simulink model "foc_model"  (R2020b)
settings: Solver=VariableStepAuto  StartTime=0.0  StopTime=0.08  FixedStep=tsim  RelTol=1e-3
undefined symbols (not defined in the file): denZC_id, denZC_iq, denZC_w, ee_sli_rtmsupport, gcbh, numZC_id, numZC_iq, numZC_w, torque0, Tsc
libraries: fl_lib x32, ee_lib x23, nesl_utility x15, slctrlblks x3, eeDiscretePi x3, eeTransforms x2, eeDqVoltageLimiter x1, eePmsmCurrentReferenceGen x1, simulink x1, eePwmGeneratorTwoLevel x1
(part 1 of 2)
settings Model: Creator=1  LastModifiedBy=ahudobin
settings SimscapeCC: SimscapeLogType=all  SimscapeLogDataHistory=10000

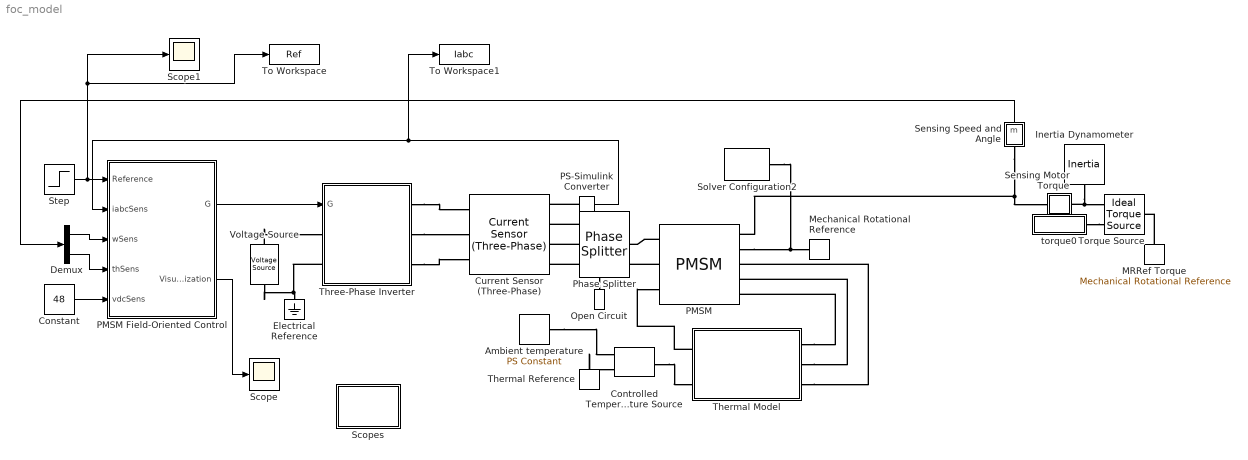
== system foc_model ==
  Ambient temperature : fl_lib/Physical Signals/Sources/PS Constant  constant=298 K
  Constant : Constant  Value=48
  Controlled Temperature Source : fl_lib/Thermal/Thermal Sources/Controlled Temperature Source
  Current Sensor (Three-Phase) : ee_lib/Sensors & Transducers/Current Sensor (Three-Phase)
      settings: InternalSimscapePortConfiguration="{\"Bottom\":[],\"Left\":[{\"id\":\"a1\",\"label\":\"a1\",\"type\":\"foundation.electrical.electrical\"},{\"id\":\"b1\",\"label\":\"b1\",\"type\":\"foundation.electrical.electrical\"},{\"id\":\"c1\",\"label\":\"c1\",\"type\":\"foundation.electrical.electrical\"}],\"Right\":[{\"id\":\"I_output\",\"label\":\"I\",\"type\":\"output\"},{\"id\":\"a2\",\"label\":\"a2\",\"type\":\"foundation.electrical.electrical\"},{\"id\":\"b2\",\"label\":\"b2\",\"type\":\"foundation.electrical.electrical\"},{\"id\":\"c2\",\"label\":\"c2\",\"type\":\"foundation.electrical.electrical\"}],\"Top\":[]}"
  Demux : Demux  Outputs=2
  Electrical Reference : fl_lib/Electrical/Electrical Elements/Electrical Reference
  Inertia Dynamometer : fl_lib/Mechanical/Rotational Elements/Inertia  inertia=1 kg*m^2  num_ports=foundation.enum.numPorts2.one  w_specify=on  w_priority=High  w=0 rpm  w_nominal_specify=off  w_nominal_unit=rad/s  w_nominal_value=1  t_specify=off  t_priority=High  t=0 N*m  t_nominal_specify=off  t_nominal_unit=N*m  t_nominal_value=1
  MRRef Torque : fl_lib/Mechanical/Rotational Elements/Mechanical Rotational Reference
  Mechanical Rotational Reference : fl_lib/Mechanical/Rotational Elements/Mechanical Rotational Reference
  Open Circuit : fl_lib/Electrical/Electrical Elements/Open Circuit  v_specify=off  v_priority=None  v=0 V  v_nominal_specify=off  v_nominal_unit=V  v_nominal_value=1
      settings: SourceProductBaseCode=SS
  PMSM : ee_lib/Electromechanical/Permanent Magnet/PMSM  winding_type=ee.enum.statorconnection.wye  machine_param=ee.enum.pmsm.parameterization.constant  nPolePairs=N  pmflux_param=ee.enum.pmflux.fluxlinkage  pm_flux_linkage=PM Wb  torque_constant=0.18 N*m/A  back_emf_constant=0.18 V/(rad/s)  stator_param=ee.enum.statorparam.LdLqL0  Ld=Ld H  Lq=Lq H  idVec=[-200, 0, 200] A  iqVec=[-200, 0, 200] A  LdMatrix=0.0002 * ones(3, 3) H  LqMatrix=0.0002 * ones(3, 3) H  PmMatrix=0.1 * ones(3, 3) Wb  ktMatrix=0.18 * ones(3, 3) N*m/A  keMatrix=0.18 * ones(3, 3) V/(rad/s)  L0=L0 H  Ls=0.0002 H  Lm=-0.00002 H  Ms=0.00002 H  Rs=Rs Ohm  zero_sequence=ee.enum.park.zerosequence.include  J=0.252 kg*m^2  lam=0 N*m/(rad/s)  axes_param=ee.enum.rotorangle.daxis  i_d_specify=off  i_d_priority=None  i_d=0 A  i_d_nominal_specify=off  i_d_nominal_unit=A  i_d_nominal_value=1  i_q_specify=off  i_q_priority=None  i_q=0 A  i_q_nominal_specify=off  i_q_nominal_unit=A  i_q_nominal_value=1  torque_specify=off  torque_priority=None  torque=0 N*m  torque_nominal_specify=off  torque_nominal_unit=N*m  torque_nominal_value=1  angular_velocity_specify=off  angular_velocity_priority=High  angular_velocity=0 rpm  angular_velocity_nominal_specify=off  angular_velocity_nominal_unit=rpm  angular_velocity_nominal_value=1  angular_position_specify=off  angular_position_priority=High  angular_position=0 deg  angular_position_nominal_specify=off  angular_position_nominal_unit=deg  angular_position_nominal_value=1  loss_param=ee.enum.ironloss.none  losses_oc=[0, 0, 0] W  losses_sc=[0, 0, 0] W  f_losses=60 Hz  Isc_losses=95 A  Tmeas=298.15 K  alpha=3.93e-3 1/K  alpha_flux=-0.001 1/K  stator_thermal_mass=100 J/K  rotor_thermal_mass=200 J/K  Rm_percent_rotor=90  Rd_percent_rotor=30  temperatureA_specify=off  temperatureA_priority=High  temperatureA=25 degC  temperatureA_nominal_specify=off  temperatureA_nominal_unit=degC  temperatureA_nominal_value=1  temperatureB_specify=off  temperatureB_priority=High  temperatureB=25 degC  temperatureB_nominal_specify=off  temperatureB_nominal_unit=degC  temperatureB_nominal_value=1  temperatureC_specify=off  temperatureC_priority=High  temperatureC=25 degC  temperatureC_nominal_specify=off  temperatureC_nominal_unit=degC  temperatureC_nominal_value=1  temperatureR_specify=off  temperatureR_priority=High  temperatureR=25 degC  temperatureR_nominal_specify=off  temperatureR_nominal_unit=degC  temperatureR_nominal_value=1
      settings: InternalSimscapePortConfiguration="{\"Bottom\":[],\"Left\":[{\"id\":\"N\",\"label\":\"~\",\"type\":\"foundation.electrical.three_phase\"},{\"id\":\"n\",\"label\":\"n\",\"type\":\"foundation.electrical.electrical\"},{\"id\":\"HR\",\"label\":\"HR\",\"type\":\"foundation.thermal.thermal\"}],\"Right\":[{\"id\":\"R\",\"label\":\"R\",\"type\":\"foundation.mechanical.rotational.rotational\"},{\"id\":\"C\",\"label\":\"C\",\"type\":\"foundation.mechanical.rotational.rotational\"},{\"id\":\"HA\",\"label\":\"HA\",\"type\":\"foundation.thermal.thermal\"},{\"id\":\"HB\",\"label\":\"HB\",\"type\":\"foundation.thermal.thermal\"},{\"id\":\"HC\",\"label\":\"HC\",\"type\":\"foundation.thermal.thermal\"}],\"Top\":[]}"
  PMSM Field-Oriented Control : Subsystem  AncestorBlock=eePmsmFieldOrientedControl/PMSM Field-Oriented Control  LoadFcn=ee_sli_rtmsupport( 'loadfcn', gcbh );  mask(PMSM Field-Oriented Control){winding_type=Wye-wound, CtrlMode=Torque control, Vnom=48, Pmax=700, Tmax=15, p=15, Vdc_on=24, Ts=5e-6, Tsc=1e-4, CtrlType=PI control, Kp_w=1, Ki_w=1, Kv_w=1, Kaw_w=1, RefType=Zero d-axis control, rpmVec=[0, 3000], TqVec=[-100, 0, 100], VdcVec=[300, 350], PWMMode=SVM: space vector modulation, ModFactor=1, idMatrix=zeros(2,3,2), iqMatrix=zeros(2,3,2), psim=0.04, Ld=0.00024, Lq=0.00029, Rs=0.01, AxisAlignment=Q-axis, Kp_id=1.6833825332468, Ki_id=35.616822421664, Kaw_id=1, Kp_iq=0.3671, Ki_iq=21.87, Kaw_iq=1, AxisPrio=Q-axis, ActZC=off, ActFF=on, ParamTypeFF=Constant parameters, LdFF=0.00024, LqFF=0.00029, psimFF=0.04, idVect=[-200, 0, 200], iqVect=[-200, 0, 200], LdMatrix=0.0002 * ones(3, 3), LqMatrix=0.0002 * ones(3, 3), psimMatrix=0.04 * ones(3, 3), CPWMMode=SVM: space vector modulation, SamplingMode=Natural, fsw=1000}
      mask prompts: winding_type "physmod:ee:library:comments:control:eePmsmFieldOrientedControl:WindingType_MP"; CtrlMode "physmod:ee:library:comments:control:eePmsmFieldOrientedControl:ControlMode_MP"; Vnom "physmod:ee:library:comments:control:eePmsmFieldOrientedControl:NominalDclinkVoltageV_MP"; Pmax "physmod:ee:library:comments:control:eePmsmFieldOrientedControl:MaximumPowerW_MP"; Tmax "physmod:ee:library:comments:control:eePmsmFieldOrientedControl:MaximumTorqueNm_MP"; p "physmod:ee:library:comments:control:eePmsmFieldOrientedControl:NumberOfRotorPolePairs_MP"; Vdc_on "physmod:ee:library:comments:control:eePmsmFieldOrientedControl:InverterDclinkVoltageThresholdV_MP"; Ts "physmod:ee:library:comments:control:eePmsmFieldOrientedControl:FundamentalSampleTimes_MP"; Tsc "physmod:ee:library:comments:control:eePmsmFieldOrientedControl:ControlSampleTimes_MP"; CtrlType "physmod:ee:library:comments:control:eePmsmFieldOrientedControl:ControlType_MP"; Kp_w "physmod:ee:library:comments:control:eePmsmFieldOrientedControl:ControllerProportionalGain_MP"; Ki_w "physmod:ee:library:comments:control:eePmsmFieldOrientedControl:ControllerIntegralGain_MP"; Kv_w "physmod:ee:library:comments:control:eePmsmFieldOrientedControl:PControllerProportionalGain_MP"; Kaw_w "physmod:ee:library:comments:control:eePmsmFieldOrientedControl:IntegralAntiwindupGain_MP"; RefType "physmod:ee:library:comments:control:eePmsmFieldOrientedControl:CurrentReferences_MP"; rpmVec "physmod:ee:library:comments:control:eePmsmFieldOrientedControl:MechanicalSpeedVectorWMechanicalrpm_MP"; TqVec "physmod:ee:library:comments:control:eePmsmFieldOrientedControl:TorqueReferenceVectorTqRefNm_MP"; VdcVec "physmod:ee:library:comments:control:eePmsmFieldOrientedControl:DClinkVoltageVectorVdcV_MP"; PWMMode "physmod:ee:library:comments:control:eePmsmCurrentReferenceGen:PWMMethod_MP"; ModFactor "physmod:ee:library:comments:control:eePmsmCurrentReferenceGen:ModulationFactor_MP"; idMatrix "physmod:ee:library:comments:control:eePmsmFieldOrientedControl:DaxisCurrentReferenceMatrixIdwMechanicalTqRefVdcA_MP"; iqMatrix "physmod:ee:library:comments:control:eePmsmFieldOrientedControl:QaxisCurrentReferenceMatrixIqwMechanicalTqRefVdcA_MP"; psim "physmod:ee:library:comments:control:eePmsmFieldOrientedControl:PermanentMagnetFluxLinkageWb_MP"; Ld "physmod:ee:library:comments:control:eePmsmFieldOrientedControl:DaxisInductanceH_MP"; Lq "physmod:ee:library:comments:control:eePmsmFieldOrientedControl:QaxisInductanceH_MP"; Rs "physmod:ee:library:comments:control:eePmsmFieldOrientedControl:StatorResistanceOhm_MP"; AxisAlignment "physmod:ee:library:comments:control:eePmsmFieldOrientedControl:PhaseaAxisAlignment_MP"; Kp_id "physmod:ee:library:comments:control:eePmsmFieldOrientedControl:DaxisCurrentProportionalGain_MP"; Ki_id "physmod:ee:library:comments:control:eePmsmFieldOrientedControl:DaxisCurrentIntegralGain_MP"; Kaw_id "physmod:ee:library:comments:control:eePmsmFieldOrientedControl:DaxisCurrentAntiwindupGain_MP"; Kp_iq "physmod:ee:library:comments:control:eePmsmFieldOrientedControl:QaxisCurrentProportionalGain_MP"; Ki_iq "physmod:ee:library:comments:control:eePmsmFieldOrientedControl:QaxisCurrentIntegralGain_MP"; Kaw_iq "physmod:ee:library:comments:control:eePmsmFieldOrientedControl:QaxisCurrentAntiwindupGain_MP"; AxisPrio "physmod:ee:library:comments:control:eePmsmFieldOrientedControl:AxisPrioritization_MP"; ActZC "physmod:ee:library:comments:control:eePmsmFieldOrientedControl:EnableZeroCancellation_MP"; ActFF "physmod:ee:library:comments:control:eePmsmFieldOrientedControl:EnablePrecontrolVoltage_MP"; ParamTypeFF "physmod:ee:library:comments:control:eePmsmFieldOrientedControl:MachineParameters_MP"; LdFF "physmod:ee:library:comments:control:eePmsmFieldOrientedControl:DaxisInductanceForFeedforwardPrecontrolH_MP"; LqFF "physmod:ee:library:comments:control:eePmsmFieldOrientedControl:QaxisInductanceForFeedforwardPrecontrolH_MP"; psimFF "physmod:ee:library:comments:control:eePmsmFieldOrientedControl:PermanentMagnetFluxLinkageForFeedforwardPrecontrolWb_MP"; idVect "physmod:ee:library:comments:control:eePmsmFieldOrientedControl:DaxisCurrentVectorIdA_MP"; iqVect "physmod:ee:library:comments:control:eePmsmFieldOrientedControl:QaxisCurrentVectorIqA_MP"; LdMatrix "physmod:ee:library:comments:control:eePmsmFieldOrientedControl:LdMatrixLdidiqH_MP"; LqMatrix "physmod:ee:library:comments:control:eePmsmFieldOrientedControl:LqMatrixLqidiqH_MP"; psimMatrix "physmod:ee:library:comments:control:eePmsmFieldOrientedControl:PermanentMagnetFluxLinkageMatrixPMidiqWb_MP"; CPWMMode "physmod:ee:library:comments:control:eePmsmFieldOrientedControl:PWMMethod_MP"; SamplingMode "physmod:ee:library:comments:control:eePmsmFieldOrientedControl:SamplingMode_MP"; fsw "physmod:ee:library:comments:control:eePmsmFieldOrientedControl:SwitchingFrequencyHz_MP"
      mask help: physmod:ee:library:comments:control:eePmsmFieldOrientedControl:PMSMFieldOrientedControl_MD
      mask init:
      | if ParamTypeFF == 1
      |     idVect = [-200, 200];
      |     iqVect = [-200, 200];
      |     LdMatrix = LdFF*ones(2, 2);
      |     LqMatrix = LqFF*ones(2, 2);
      |     psimMatrix = psimFF*ones(2, 2);
      | end
      | 
      | switch winding_type
      |     case 1
      |         theta_offset = 0;
      |     case 2
      |         theta_offset = -(120/p)*pi/180;
      |     otherwise
      |         theta_offset = 0;
      | end
      | 
      | switch CPWMMode
      |     case 'SPWM: sinusoidal PWM'
      |         set_param(gcb,'PWMMode','SPWM: sinusoidal PWM');
      |     case 'SVM: space vector modulation'
      |         set_param(gcb,'PWMMode','SVM: space vector modulation')
      | end
      settings: CopyFcn=ee_sli_rtmsupport( 'copyfcn', gcbh );  DeleteFcn=ee_sli_rtmsupport( 'deletefcn', gcbh );  ModelCloseFcn=ee_sli_rtmsupport( 'modelclosefcn', gcbh );  PostSaveFcn=ee_sli_rtmsupport( 'postsavefcn', gcbh );  PreCopyFcn=ee_sli_rtmsupport( 'precopyfcn', gcbh );  OpenFcn=ee_sli_rtmsupport( 'openfcn', gcbh );  CloseFcn=ee_sli_rtmsupport( 'closefcn', gcbh );  PreDeleteFcn=ee_sli_rtmsupport( 'predeletefcn', gcbh );
      mask Help: web(nesl_help(gcbh))
      mask TypeOptions winding_type: physmod:ee:library:comments:control:eePmsmFieldOrientedControl:WyeWound_PV | physmod:ee:library:comments:control:eePmsmFieldOrientedControl:DeltaWound_PV
      mask Callback winding_type: ee.mask.callbackPopupPmsmFoc(gcb);
      mask TypeOptions CtrlMode: physmod:ee:library:comments:control:eePmsmFieldOrientedControl:VelocityControl_PV | physmod:ee:library:comments:control:eePmsmFieldOrientedControl:TorqueControl_PV
      mask Callback CtrlMode: ee.mask.callbackPopupPmsmFoc(gcb);
      mask TypeOptions Vnom:
      | Outer loop control/PMSM Current Reference
      | Generator/Vnom
      mask TypeOptions Pmax:
      | Outer loop control/PMSM Current Reference
      | Generator/Pmax
      mask TypeOptions Tmax:
      | Outer loop control/PMSM Current Reference
      | Generator/Tmax
      mask TypeOptions CtrlType: Outer loop control/Velocity Controller/CtrlType
      mask Callback CtrlType: ee.mask.callbackPopupPmsmFoc(gcb);
      mask TypeOptions Kp_w: Outer loop control/Velocity Controller/Kp_w
      mask TypeOptions Ki_w: Outer loop control/Velocity Controller/Ki_w
      mask TypeOptions Kv_w: Outer loop control/Velocity Controller/Kv_w
      mask TypeOptions Kaw_w: Outer loop control/Velocity Controller/Kaw_w
      mask TypeOptions RefType:
      | Outer loop control/PMSM Current Reference
      | Generator/RefType
      mask Callback RefType: ee.mask.callbackPopupPmsmFoc(gcb);
      mask TypeOptions rpmVec:
      | Outer loop control/PMSM Current Reference
      | Generator/rpmVec
      mask TypeOptions TqVec:
      | Outer loop control/PMSM Current Reference
      | Generator/TqVec
      mask TypeOptions VdcVec:
      | Outer loop control/PMSM Current Reference
      | Generator/VdcVec
      mask TypeOptions PWMMode:
      | Outer loop control/PMSM Current Reference
      | Generator/PWMMode
      mask TypeOptions ModFactor:
      | Outer loop control/PMSM Current Reference
      | Generator/ModFactor
      mask TypeOptions idMatrix:
      | Outer loop control/PMSM Current Reference
      | Generator/idMatrix
      mask TypeOptions iqMatrix:
      | Outer loop control/PMSM Current Reference
      | Generator/iqMatrix
      mask TypeOptions psim:
      | Outer loop control/PMSM Current Reference
      | Generator/psim
      mask TypeOptions Ld:
      | Outer loop control/PMSM Current Reference
      | Generator/Ld
      mask TypeOptions Lq:
      | Outer loop control/PMSM Current Reference
      | Generator/Lq
      mask TypeOptions Rs:
      | Outer loop control/PMSM Current Reference
      | Generator/Rs
      mask TypeOptions AxisAlignment: Inner loop control/Park Transform/AxisAlignment
      mask TypeOptions Kp_id:
      | Inner loop control/PMSM Current Controller
      | with Pre-Control/Kp_id
      mask TypeOptions Ki_id:
      | Inner loop control/PMSM Current Controller
      | with Pre-Control/Ki_id
      mask TypeOptions Kaw_id:
      | Inner loop control/PMSM Current Controller
      | with Pre-Control/Kaw_id
      mask TypeOptions Kp_iq:
      | Inner loop control/PMSM Current Controller
      | with Pre-Control/Kp_iq
      mask TypeOptions Ki_iq:
      | Inner loop control/PMSM Current Controller
      | with Pre-Control/Ki_iq
      mask TypeOptions Kaw_iq:
      | Inner loop control/PMSM Current Controller
      | with Pre-Control/Kaw_iq
      mask TypeOptions AxisPrio:
      | Inner loop control/PMSM Current Controller
      | with Pre-Control/AxisPrio
      mask TypeOptions ActZC:
      | Inner loop control/PMSM Current Controller
      | with Pre-Control/ActZC
      mask TypeOptions ActFF:
      | Inner loop control/PMSM Current Controller
      | with Pre-Control/ActFF
      mask Callback ActFF: ee.mask.callbackPopupPmsmFoc(gcb);
      mask TypeOptions ParamTypeFF: physmod:ee:library:comments:control:eePmsmFieldOrientedControl:ConstantParameters_PV | physmod:ee:library:comments:control:eePmsmFieldOrientedControl:LookupTableBasedParameters_PV
      mask Callback ParamTypeFF: ee.mask.callbackPopupPmsmFoc(gcb);
      mask TypeOptions idVect:
      | Inner loop control/PMSM Current Controller
      | with Pre-Control/idVect
      mask TypeOptions iqVect:
      | Inner loop control/PMSM Current Controller
      | with Pre-Control/iqVect
      mask TypeOptions LdMatrix:
      | Inner loop control/PMSM Current Controller
      | with Pre-Control/LdMatrix
      mask TypeOptions LqMatrix:
      | Inner loop control/PMSM Current Controller
      | with Pre-Control/LqMatrix
      mask TypeOptions psimMatrix:
      | Inner loop control/PMSM Current Controller
      | with Pre-Control/psimMatrix
      mask TypeOptions CPWMMode:
      | PWM/PWM Generator
      | (Three-phase, Two-level)/CPWMMode
      mask TypeOptions SamplingMode:
      | PWM/PWM Generator
      | (Three-phase, Two-level)/SamplingMode
      mask DialogControl Container4 Prompt: physmod:ee:library:comments:control:eePmsmFieldOrientedControl:tab_General
      mask DialogControl winding_type Prompt: Winding type
      mask DialogControl CtrlMode Prompt: Control mode
      mask DialogControl Vnom Prompt: Nominal dc-link voltage (V)
      mask DialogControl Pmax Prompt: Maximum power (W)
      mask DialogControl Tmax Prompt: Maximum torque (N*m)
      mask DialogControl p Prompt: Number of rotor pole pairs
      mask DialogControl Vdc_on Prompt: Inverter dc-link voltage threshold (V)
      mask DialogControl Ts Prompt: Fundamental sample time (s)
      mask DialogControl Tsc Prompt: Control sample time (s)
      mask DialogControl Container7 Prompt: physmod:ee:library:comments:control:eePmsmFieldOrientedControl:tab_OuterLoop
      mask DialogControl CtrlType Prompt: Control type
      mask DialogControl Kp_w Prompt: Controller proportional gain
      mask DialogControl Ki_w Prompt: Controller integral gain
      mask DialogControl Kv_w Prompt: P controller proportional gain
      mask DialogControl Kaw_w Prompt: Integral anti-windup gain
      mask DialogControl RefType Prompt: Current references
      mask DialogControl rpmVec Prompt: Mechanical speed vector, wMechanical (rpm)
      mask DialogControl TqVec Prompt: Torque reference vector, TqRef (N*m)
      mask DialogControl VdcVec Prompt: DC-link voltage vector, Vdc (V)
      mask DialogControl PWMMode Prompt: PWM method
      mask DialogControl ModFactor Prompt: Modulation factor
      mask DialogControl idMatrix Prompt: D-axis current reference matrix, id(wMechanical,TqRef,Vdc), (A)
      mask DialogControl iqMatrix Prompt: Q-axis current reference matrix, iq(wMechanical,TqRef,Vdc), (A)
      mask DialogControl psim Prompt: Permanent magnet flux linkage (Wb)
      mask DialogControl Ld Prompt: D-axis inductance (H)
      mask DialogControl Lq Prompt: Q-axis inductance (H)
      mask DialogControl Rs Prompt: Stator resistance (Ohm)
      mask DialogControl Container8 Prompt: physmod:ee:library:comments:control:eePmsmFieldOrientedControl:tab_InnerLoop
      mask DialogControl AxisAlignment Prompt: Phase-a axis alignment
      mask DialogControl Kp_id Prompt: D-axis current proportional gain
      mask DialogControl Ki_id Prompt: D-axis current integral gain
      mask DialogControl Kaw_id Prompt: D-axis current anti-windup gain
      mask DialogControl Kp_iq Prompt: Q-axis current proportional gain
      mask DialogControl Ki_iq Prompt: Q-axis current integral gain
      mask DialogControl Kaw_iq Prompt: Q-axis current anti-windup gain
      mask DialogControl AxisPrio Prompt: Axis prioritization
      mask DialogControl ActZC Prompt: Enable zero cancellation
      mask DialogControl ActFF Prompt: Enable pre-control voltage
      mask DialogControl ParamTypeFF Prompt: Machine parameters
      mask DialogControl LdFF Prompt: D-axis inductance for feed-forward pre-control (H)
      mask DialogControl LqFF Prompt: Q-axis inductance for feed-forward pre-control (H)
      mask DialogControl psimFF Prompt: Permanent magnet flux linkage for feed-forward pre-control (Wb)
      mask DialogControl idVect Prompt: D-axis current vector, id (A)
      mask DialogControl iqVect Prompt: Q-axis current vector, iq (A)
      mask DialogControl LdMatrix Prompt: Ld matrix, Ld(id,iq), (H)
      mask DialogControl LqMatrix Prompt: Lq matrix, Lq(id,iq), (H)
      mask DialogControl psimMatrix Prompt: Permanent magnet flux linkage matrix, PM(id,iq), (Wb)
      mask DialogControl Container9 Prompt: physmod:ee:library:comments:control:eePmsmFieldOrientedControl:tab_PWM
      mask DialogControl CPWMMode Prompt: PWM method
      mask DialogControl SamplingMode Prompt: Sampling mode
      mask DialogControl fsw Prompt: Switching frequency (Hz)
  PS-Simulink Converter : nesl_utility/PS-Simulink Converter  PhysicalDomain=network_engine_domain  SubClassName=ps_output  LeftPortType=input  RightPortType=output  PseudoPeriodic=off  Frequencies=[]  Unit=inherit  AffineConversion=off
  Phase Splitter : ee_lib/Connectors & References/Phase Splitter
      settings: SourceProductBaseCode=PS
  Scope : Scope
  Scope1 : Scope
  Scopes : Subsystem
  Sensing Motor Torque : Subsystem
      mask Display: disp('trq');
  Sensing Speed and Angle : Subsystem
      mask Display: disp('m')
  Solver Configuration2 : nesl_utility/Solver Configuration  PhysicalDomain=network_engine_domain  SubClassName=solver  LeftPortType=input  RightPortType=generic  Tones=[]  Harmonics=[]  SimulateNoise=off  Profile=off  UseLocalSampling=off  EnableSwitchedLinearOptims=on  FrequencyDomain=off  UseCCode=off  RelTol=0.001  AbsTol=1e-06  MinStep=1e-09  ToWorkspace=off  RevertToSquareIcSolve=off  NumHomotopyIterations=100  PhasorMode=off  PhasorModeNumHarmonics=1  DoDC=off  ResidualTolerance=1e-09  UseLocalSolver=off  LocalSolverChoice=NE_BACKWARD_EULER_ADVANCER  LocalSolverSampleTime=0.001  DoFixedCost=off  MaxNonlinIter=3  MaxModeIter=2  ComputeImpulses=off  ImpulseIterations=2  LinearAlgebra=auto  EquationFormulation=NE_TIME_EF  DelaysMemoryBudget=1024  AutomaticFiltering=on  FilteringTimeConstant=0.001  PartitionStorageMethod=AS_NEEDED  PartitionMemoryBudget=1024  PartitionMethod=ROBUST
  Step : Step  Time=0.05  After=15  SampleTime=Tsc
  Thermal Model : Subsystem
  Thermal Reference : fl_lib/Thermal/Thermal Elements/Thermal Reference
  Three-Phase Inverter : Subsystem  Tag=PublishSubsystem
  To Workspace : ToWorkspace  VariableName=Ref  SaveFormat=Structure With Time  SampleTime=Tsc
  To Workspace1 : ToWorkspace  VariableName=Iabc  SampleTime=Tsc
  Torque Source : fl_lib/Mechanical/Mechanical Sources/Ideal Torque Source
  Voltage Source : ee_lib/Sources/Voltage Source  dc_voltage=48 V  ac_voltage=0 V  ac_shift=0 rad  ac_frequency=0 Hz  noise_mode=0  PSD=0 V^2/Hz  repeatability=1  auto_seed=789877936  user_seed=0  sample_time=1e-3 s  i_specify=off  i_priority=None  i=0 A  i_nominal_specify=off  i_nominal_unit=A  i_nominal_value=1  v_specify=off  v_priority=None  v=0 V  v_nominal_specify=off  v_nominal_unit=V  v_nominal_value=1
  torque0 : Subsystem
      mask Display: disp('torque0');
  wires:
  Constant/1 -> PMSM Field-Oriented Control/5(vdcSens)
  Step/1 -> To Workspace/1, Scope1/1, PMSM Field-Oriented Control/1(Reference)
  PMSM Field-Oriented Control/1(G) -> Three-Phase Inverter/1(G)
  PS-Simulink Converter/1 -> To Workspace1/1, PMSM Field-Oriented Control/2(iabcSens)
  PMSM Field-Oriented Control/2(Visualization) -> Scope/1
  Sensing Speed and Angle/1(m) -> Demux/1
  Demux/1 -> PMSM Field-Oriented Control/3(wSens)
  Demux/2 -> PMSM Field-Oriented Control/4(thSens)
  connections:
  Three-Phase Inverter/RConn1 -- Current Sensor (Three-Phase)/LConn1
  Three-Phase Inverter/RConn2 -- Current Sensor (Three-Phase)/LConn2
  Three-Phase Inverter/RConn3 -- Current Sensor (Three-Phase)/LConn3
  Phase Splitter/RConn1 -- Current Sensor (Three-Phase)/RConn2
  Phase Splitter/RConn2 -- Current Sensor (Three-Phase)/RConn3
  Phase Splitter/RConn3 -- Current Sensor (Three-Phase)/RConn4
  PMSM/LConn1 -- Phase Splitter/LConn1
  PS-Simulink Converter/LConn1 -- Current Sensor (Three-Phase)/RConn1
  Voltage Source/LConn1 -- Three-Phase Inverter/LConn1
  Voltage Source/RConn1 -- Three-Phase Inverter/LConn2 -- Electrical Reference/LConn1
  Ambient temperature/RConn1 -- Controlled Temperature Source/RConn1
  Thermal Reference/LConn1 -- Controlled Temperature Source/RConn2
  Controlled Temperature Source/LConn1 -- Thermal Model/LConn2
  Thermal Model/LConn1 -- PMSM/LConn3
  PMSM/LConn2 -- Open Circuit/LConn1
  Thermal Model/RConn3 -- PMSM/RConn3
  Thermal Model/RConn2 -- PMSM/RConn4
  Thermal Model/RConn1 -- PMSM/RConn5
  PMSM/RConn2 -- Solver Configuration2/RConn1 -- Mechanical Rotational Reference/LConn1
  Sensing Speed and Angle/LConn1 -- Sensing Motor Torque/LConn1 -- PMSM/RConn1
  Sensing Motor Torque/RConn1 -- Torque Source/RConn2 -- Inertia Dynamometer/LConn1
  MRRef Torque/LConn1 -- Torque Source/LConn1
  torque0/RConn1 -- Torque Source/RConn1

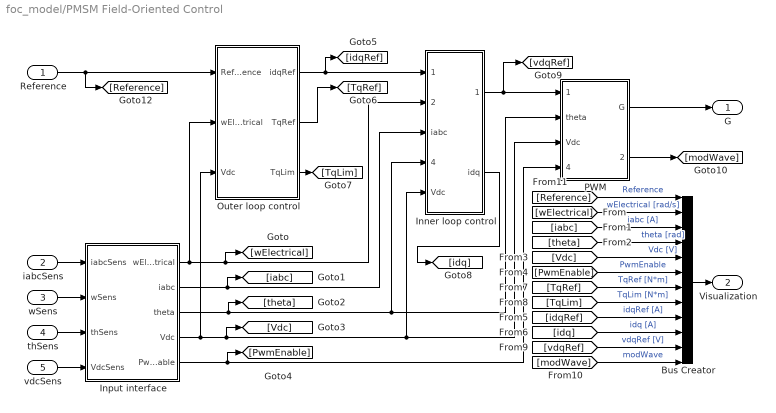
== system foc_model/PMSM Field-Oriented Control ==
  Reference : Inport  SampleTime=Tsc
  iabcSens : Inport  Port=2  SampleTime=Tsc
  wSens : Inport  Port=3  SampleTime=Tsc
  thSens : Inport  Port=4  SampleTime=Tsc
  vdcSens : Inport  Port=5  SampleTime=Tsc
  Bus Creator : BusCreator  Inputs=12
  Inner loop control : Subsystem
  Input interface : Subsystem
  Outer loop control : Subsystem
  PWM : Subsystem
  G : Outport  VectorParamsAs1DForOutWhenUnconnected=off
  Visualization : Outport  Port=2  VectorParamsAs1DForOutWhenUnconnected=off
  wires:
  [modWave] -> Bus Creator/12  "modWave"
  [vdqRef] -> Bus Creator/11  "vdqRef [V]"
  [idq] -> Bus Creator/10  "idq [A]"
  [idqRef] -> Bus Creator/9  "idqRef [A]"
  [TqLim] -> Bus Creator/8  "TqLim [N*m]"
  [TqRef] -> Bus Creator/7  "TqRef [N*m]"
  [PwmEnable] -> Bus Creator/6  "PwmEnable"
  [Vdc] -> Bus Creator/5  "Vdc [V]"
  [theta] -> Bus Creator/4  "theta [rad]"
  [iabc] -> Bus Creator/3  "iabc [A]"
  [wElectrical] -> Bus Creator/2  "wElectrical [rad/s]"
  [Reference] -> Bus Creator/1  "Reference"
  PWM/2(ModWave) -> [modWave]
  Inner loop control/2(idq) -> [idq]
  Outer loop control/3(TqLim) -> [TqLim]
  Outer loop control/2(TqRef) -> [TqRef]
  Bus Creator/1 -> Visualization/1
  PWM/1(G) -> G/1
  Input interface/5(PwmEnable) -> PWM/4(PwmEnable), [PwmEnable]
  Inner loop control/1(vdqRef) -> PWM/1(vdqRef), [vdqRef]
  Input interface/1(wElectrical) -> Outer loop control/2(wElectrical), Inner loop control/2(wElectrical), [wElectrical]
  Input interface/4(Vdc) -> Outer loop control/3(Vdc), Inner loop control/5(Vdc), PWM/3(Vdc), [Vdc]
  Reference/1 -> Outer loop control/1(Reference), [Reference]
  vdcSens/1 -> Input interface/4(VdcSens)
  thSens/1 -> Input interface/3(thSens)
  wSens/1 -> Input interface/2(wSens)
  iabcSens/1 -> Input interface/1(iabcSens)
  Outer loop control/1(idqRef) -> Inner loop control/1(idq_ref), [idqRef]
  Input interface/3(theta) -> Inner loop control/4(theta), PWM/2(theta), [theta]
  Input interface/2(iabc) -> Inner loop control/3(iabc), [iabc]

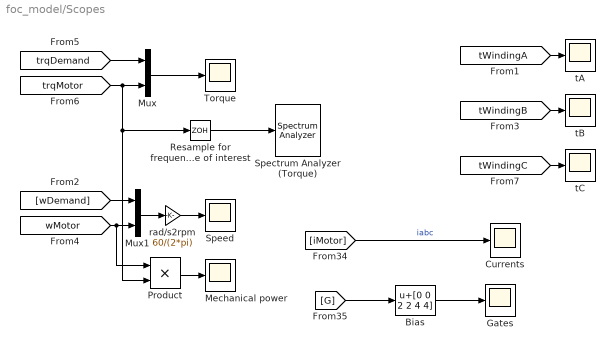
== system foc_model/Scopes ==
  Bias : Bias  Bias=[0 0 2 2 4 4]
  Currents : Scope
  Gates : Scope
  Mechanical power : Scope
  Mux : Mux  Inputs=2
  Mux1 : Mux  Inputs=2
  Product : Product
  Resample for frequency range of interest : ZeroOrderHold  SampleTime=2.5e-5
  Spectrum Analyzer (Torque) : SpectrumAnalyzer  Tag=PublishScope
  Speed : Scope
  Torque : Scope
  rad/s2rpm : Gain  Gain=60/(2*pi)
  tA : Scope
  tB : Scope
  tC : Scope
  wires:
  rad/s2rpm/1 -> Speed/1
  Mux/1 -> Torque/1
  [iMotor] -> Currents/1  "iabc"
  [trqDemand] -> Mux/1
  [wDemand] -> Mux1/1
  Mux1/1 -> rad/s2rpm/1
  [trqMotor] -> Product/2, Resample for frequency range of interest/1, Mux/2
  [wMotor] -> Product/1, Mux1/2
  [G] -> Bias/1
  Bias/1 -> Gates/1
  Product/1 -> Mechanical power/1
  Resample for frequency range of interest/1 -> Spectrum Analyzer (Torque)/1
  [tWindingA] -> tA/1
  [tWindingB] -> tB/1
  [tWindingC] -> tC/1

== system foc_model/Sensing Motor Torque ==
  Ideal Torque Sensor : fl_lib/Mechanical/Mechanical Sensors/Ideal Torque Sensor
  PS-Simulink Converter2 : nesl_utility/PS-Simulink Converter  PhysicalDomain=network_engine_domain  SubClassName=ps_output  LeftPortType=input  RightPortType=output  PseudoPeriodic=off  Frequencies=[]  Unit=N*m  AffineConversion=off
  R : PMIOPort  Side=Left
  C : PMIOPort  Port=2  Side=Right
  tag scope: trqMotor=global
  wires:
  PS-Simulink Converter2/1 -> [trqMotor]
  connections:
  Ideal Torque Sensor/RConn2 -- PS-Simulink Converter2/LConn1
  R/RConn1 -- Ideal Torque Sensor/LConn1
  Ideal Torque Sensor/RConn1 -- C/RConn1

== system foc_model/Sensing Speed and Angle ==
  Ideal Rotational Motion Sensor : fl_lib/Mechanical/Mechanical Sensors/Ideal Rotational Motion Sensor  wrap_angle=simscape.enum.onoff.off  offset=0 deg
  MRRef : fl_lib/Mechanical/Rotational Elements/Mechanical Rotational Reference
  Mux : Mux  Inputs=2
  PS-Simulink Converter : nesl_utility/PS-Simulink Converter  PhysicalDomain=network_engine_domain  SubClassName=ps_output  LeftPortType=input  RightPortType=output  PseudoPeriodic=off  Frequencies=[]  Unit=rad/s  AffineConversion=off
  PS-Simulink Converter1 : nesl_utility/PS-Simulink Converter  PhysicalDomain=network_engine_domain  SubClassName=ps_output  LeftPortType=input  RightPortType=output  PseudoPeriodic=off  Frequencies=[]  Unit=rad  AffineConversion=off
  To Workspace1 : ToWorkspace  VariableName=Amot  SampleTime=Tsc
  To Workspace2 : ToWorkspace  VariableName=Wmot  SampleTime=Tsc
  R : PMIOPort  Side=Left
  m : Outport  VectorParamsAs1DForOutWhenUnconnected=off
  tag scope: wMotor=global
  wires:
  Mux/1 -> m/1
  PS-Simulink Converter/1 -> To Workspace2/1, [wMotor], Mux/1
  PS-Simulink Converter1/1 -> To Workspace1/1, Mux/2
  connections:
  Ideal Rotational Motion Sensor/RConn3 -- PS-Simulink Converter1/LConn1
  Ideal Rotational Motion Sensor/RConn1 -- MRRef/LConn1
  Ideal Rotational Motion Sensor/RConn2 -- PS-Simulink Converter/LConn1
  Ideal Rotational Motion Sensor/LConn1 -- R/RConn1

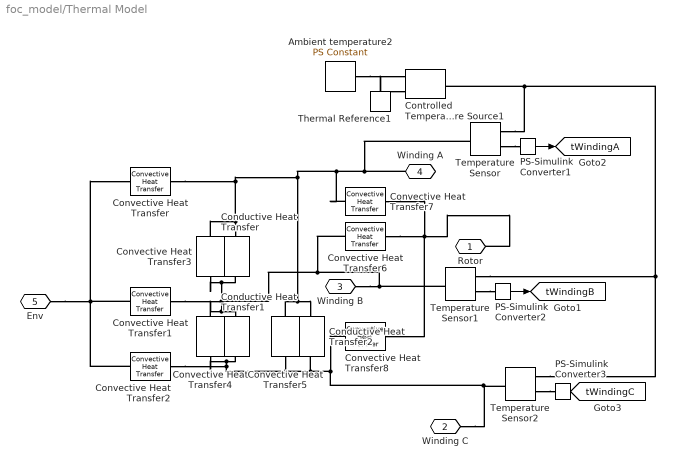
== system foc_model/Thermal Model ==
  Ambient temperature2 : fl_lib/Physical Signals/Sources/PS Constant  constant=273 K
  Conductive Heat Transfer : fl_lib/Thermal/Thermal Elements/Conductive Heat Transfer  area=1e-4 m^2  thickness=0.1 m  th_cond=401 W/(m*K)  T_specify=off  T_priority=None  T=0 K  T_nominal_specify=off  T_nominal_unit=K  T_nominal_value=1  Q_specify=off  Q_priority=None  Q=0 W  Q_nominal_specify=off  Q_nominal_unit=W  Q_nominal_value=1
  Conductive Heat Transfer1 : fl_lib/Thermal/Thermal Elements/Conductive Heat Transfer  area=1e-4 m^2  thickness=0.1 m  th_cond=401 W/(m*K)  T_specify=off  T_priority=None  T=0 K  T_nominal_specify=off  T_nominal_unit=K  T_nominal_value=1  Q_specify=off  Q_priority=None  Q=0 W  Q_nominal_specify=off  Q_nominal_unit=W  Q_nominal_value=1
  Conductive Heat Transfer2 : fl_lib/Thermal/Thermal Elements/Conductive Heat Transfer  area=1e-4 m^2  thickness=0.1 m  th_cond=401 W/(m*K)  T_specify=off  T_priority=None  T=0 K  T_nominal_specify=off  T_nominal_unit=K  T_nominal_value=1  Q_specify=off  Q_priority=None  Q=0 W  Q_nominal_specify=off  Q_nominal_unit=W  Q_nominal_value=1
  Controlled Temperature Source1 : fl_lib/Thermal/Thermal Sources/Controlled Temperature Source
  Convective Heat Transfer{,1..8} (9 alike) : fl_lib/Thermal/Thermal Elements/Convective Heat Transfer  area=1e-4 m^2  heat_tr_coeff=20 W/(m^2 * K)  T_specify=off  T_priority=None  T=0 K  T_nominal_specify=off  T_nominal_unit=K  T_nominal_value=1  Q_specify=off  Q_priority=None  Q=0 W  Q_nominal_specify=off  Q_nominal_unit=W  Q_nominal_value=1
  PS-Simulink Converter1 : nesl_utility/PS-Simulink Converter  PhysicalDomain=network_engine_domain  SubClassName=ps_output  LeftPortType=input  RightPortType=output  PseudoPeriodic=off  Frequencies=[]  Unit=inherit  AffineConversion=off
  PS-Simulink Converter2 : nesl_utility/PS-Simulink Converter  PhysicalDomain=network_engine_domain  SubClassName=ps_output  LeftPortType=input  RightPortType=output  PseudoPeriodic=off  Frequencies=[]  Unit=inherit  AffineConversion=off
  PS-Simulink Converter3 : nesl_utility/PS-Simulink Converter  PhysicalDomain=network_engine_domain  SubClassName=ps_output  LeftPortType=input  RightPortType=output  PseudoPeriodic=off  Frequencies=[]  Unit=inherit  AffineConversion=off
  Temperature Sensor : fl_lib/Thermal/Thermal Sensors/Temperature Sensor
  Temperature Sensor1 : fl_lib/Thermal/Thermal Sensors/Temperature Sensor
  Temperature Sensor2 : fl_lib/Thermal/Thermal Sensors/Temperature Sensor
  Thermal Reference1 : fl_lib/Thermal/Thermal Elements/Thermal Reference
  Rotor : PMIOPort  Side=Left
  Winding C : PMIOPort  Port=2  Side=Right
  Winding B : PMIOPort  Port=3  Side=Right
  Winding A : PMIOPort  Port=4  Side=Right
  Env : PMIOPort  Port=5  Side=Left
  tag scope: tWindingA=global, tWindingB=global, tWindingC=global
  wires:
  PS-Simulink Converter1/1 -> [tWindingA]
  PS-Simulink Converter2/1 -> [tWindingB]
  PS-Simulink Converter3/1 -> [tWindingC]
  connections:
  Env/RConn1 -- Convective Heat Transfer2/RConn1 -- Convective Heat Transfer1/RConn1 -- Convective Heat Transfer/RConn1
  Convective Heat Transfer3/RConn1 -- Temperature Sensor1/LConn1 -- Winding B/RConn1 -- Convective Heat Transfer6/RConn1 -- Convective Heat Transfer1/LConn1 -- Convective Heat Transfer4/LConn1 -- Conductive Heat Transfer1/LConn1 -- Conductive Heat Transfer/RConn1
  Convective Heat Transfer5/LConn1 -- Temperature Sensor2/LConn1 -- Winding C/RConn1 -- Convective Heat Transfer8/RConn1 -- Conductive Heat Transfer2/LConn1 -- Convective Heat Transfer2/LConn1 -- Conductive Heat Transfer1/RConn1 -- Convective Heat Transfer4/RConn1
  Convective Heat Transfer3/LConn1 -- Convective Heat Transfer/LConn1 -- Temperature Sensor/LConn1 -- Winding A/RConn1 -- Convective Heat Transfer7/RConn1 -- Conductive Heat Transfer2/RConn1 -- Convective Heat Transfer5/RConn1 -- Conductive Heat Transfer/LConn1
  Convective Heat Transfer6/LConn1 -- Convective Heat Transfer8/LConn1 -- Convective Heat Transfer7/LConn1 -- Rotor/RConn1
  Thermal Reference1/LConn1 -- Controlled Temperature Source1/RConn2
  Ambient temperature2/RConn1 -- Controlled Temperature Source1/RConn1
  Temperature Sensor/RConn1 -- Temperature Sensor2/RConn1 -- Temperature Sensor1/RConn1 -- Controlled Temperature Source1/LConn1
  Temperature Sensor/RConn2 -- PS-Simulink Converter1/LConn1
  Temperature Sensor1/RConn2 -- PS-Simulink Converter2/LConn1
  Temperature Sensor2/RConn2 -- PS-Simulink Converter3/LConn1

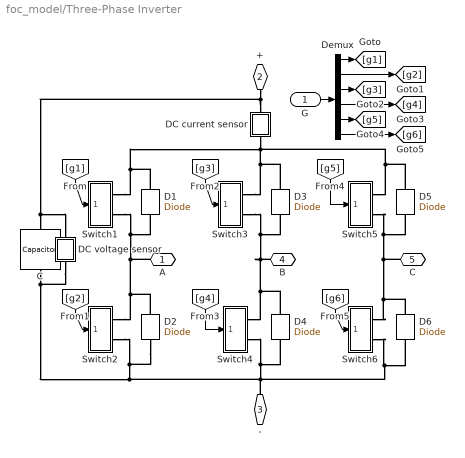
== system foc_model/Three-Phase Inverter ==
  G : Inport
  " C" : ee_lib/Passive/Capacitor  cap_option=0  c=10 F  Cvec=[ 1e-5 1e-6 ] F  Vvec=[ 0 10 ] V  CV_table_symmetry=1  f_vec=[1, 10] kHz  DFext_vec=[.8, 1.2]  C_tol=5  enable_C_tol=0  tol_distribution=1  nSigma=4  r=0.001 Ohm  g=0 1/Ohm  averaging_period=0 s  enable_operating_limits=0  operating_limit_action=2  max_working_voltage_range=[ -25 25 ] V  power_rating=1 W  enable_faults=0  fault_action=1  Cscale_faulted=100  R_faulted=0.001 Ohm  G_faulted=0 1/Ohm  tau_fault=0.001 s  enable_temporal_fault=0  t_fault=1 s  enable_behavioral_fault=0  max_permissible_voltage_range=[ -100 100 ] V  t_fail_on_voltage=1 s  i_specify=off  i_priority=Low  i=0 A  i_nominal_specify=off  i_nominal_unit=A  i_nominal_value=1  v_specify=off  v_priority=None  v=0 V  v_nominal_specify=off  v_nominal_unit=V  v_nominal_value=1  vc_specify=on  vc_priority=High  vc=500 V  vc_nominal_specify=off  vc_nominal_unit=V  vc_nominal_value=1
  D{1..6} (6 alike) : ee_lib/Semiconductors & Converters/Diode  ModelType=ee.enum.diode.modelType.exponential  IfMat=[.07, .12, .19, 1.75, 4.24, 7.32, 11.2; .16, .3, .72, 2.14, 4.02, 6.35, 9.12] A  TjVec=[25, 125] degC  VfVec=[.5, .7, .9, 1.3, 1.7, 2.1, 2.5] V  Vf=0.6 V  Ron=0.3 Ohm  Goff=1e-8 S  prmExp=2  I12=[ 0.0137 0.545 ] A  V12=[ 0.6 0.7 ] V  IS=1e-7 A  ec=1  I1=0.0137 A  V1=0.6 V  RS=0.001 Ohm  Tmeas=25 degC  N_series=1  N_parallel=1  Rz=0.3 Ohm  BV=Inf V  C_param=1  CJ=50 pF  CJ0=50 pF  VJ=1 V  Mgrad=0.5  Vvec=[ 0.1 10 100 ] V  Cvec=[ 3.5 1 0.4 ] pF  FC=0.5  Q_param=ee.enum.diode.recoveryParam.off  iRM=-7.15 A  iF=4 A  didt=-750 A/us  trr_factor=3  trr=115 ns  Qrr=1500 s*uA  TT=50 ns  tau=100 ns  T_param=1  IS_T2=1.25e-7 A  I1_T2=0.245 A  V1_T2=0.5 V  Tmeas2=125 degC  EG_param=1  EG=1.11 eV  XTI_param=1  XTI=3  dBVdT=0 V/K  Tdevice=25 degC  i_specify=off  i_priority=None  i=0 A  i_nominal_specify=off  i_nominal_unit=A  i_nominal_value=1  v_specify=off  v_priority=None  v=0 V  v_nominal_specify=off  v_nominal_unit=V  v_nominal_value=1  i_capacitor_specify=off  i_capacitor_priority=High  i_capacitor=0 A  i_capacitor_nominal_specify=off  i_capacitor_nominal_unit=A  i_capacitor_nominal_value=1  v_capacitor_specify=off  v_capacitor_priority=None  v_capacitor=0 V  v_capacitor_nominal_specify=off  v_capacitor_nominal_unit=V  v_capacitor_nominal_value=1  power_dissipated_specify=off  power_dissipated_priority=None  power_dissipated=0 W  power_dissipated_nominal_specify=off  power_dissipated_nominal_unit=W  power_dissipated_nominal_value=1  thermal_network_parameterization=ee.enum.thermalNetworkTopology.cauer  Rth=[0, 10] K/W  Rth_Foster=[4, 6] K/W  thermal_mass_parameterization=ee.enum.thermalNetwork.timeconstant  thermal_mass=[0, 1] J/K  thermal_mass_Foster=[1.5, 3] J/K  thermal_time_constant=[0, 10] s  thermal_time_constant_Foster=[6, 18] s  thermal_mass_initial_temperatures=[25, 25] degC
      settings: LogSimulationData=on
  DC current sensor : Subsystem
      mask Display: disp('i');
  DC voltage sensor : Subsystem
      mask Display: disp('v')
  Demux : Demux  Outputs=6
  Switch1 : Subsystem
  Switch2 : Subsystem
  Switch3 : Subsystem
  Switch4 : Subsystem
  Switch5 : Subsystem
  Switch6 : Subsystem
  A : PMIOPort  Tag=PMCPort  Side=Right
  + : PMIOPort  Tag=PMCPort  Port=2  Side=Left
  - : PMIOPort  Tag=PMCPort  Port=3  Side=Left
  B : PMIOPort  Tag=PMCPort  Port=4  Side=Right
  C : PMIOPort  Tag=PMCPort  Port=5  Side=Right
  wires:
  Demux/6 -> [g6]
  Demux/5 -> [g5]
  Demux/4 -> [g4]
  Demux/3 -> [g3]
  Demux/2 -> [g2]
  G/1 -> Demux/1
  Demux/1 -> [g1]
  [g1] -> Switch1/1(g)
  [g2] -> Switch2/1(g)
  [g3] -> Switch3/1(g)
  [g4] -> Switch4/1(g)
  [g5] -> Switch5/1(g)
  [g6] -> Switch6/1(g)
  connections:
  -/RConn1 -- D6/LConn1 -- Switch6/RConn2 -- Switch4/RConn2 -- D4/LConn1 -- DC voltage sensor/LConn1 -- " C"/RConn1 -- D2/LConn1 -- Switch2/RConn2
  A/RConn1 -- Switch1/RConn2 -- D1/LConn1 -- D2/RConn1 -- Switch2/RConn1
  B/RConn1 -- Switch4/RConn1 -- D4/RConn1 -- Switch3/RConn2 -- D3/LConn1
  C/RConn1 -- Switch6/RConn1 -- D6/RConn1 -- Switch5/RConn2 -- D5/LConn1
  +/RConn1 -- DC voltage sensor/RConn1 -- " C"/LConn1 -- DC current sensor/RConn1
  D3/RConn1 -- Switch3/RConn1 -- Switch1/RConn1 -- D1/RConn1 -- DC current sensor/LConn1 -- Switch5/RConn1 -- D5/RConn1

== system foc_model/torque0 ==
  Constant1 : Constant  Value=torque0
  Simulink-PS Converter : nesl_utility/Simulink-PS Converter  PhysicalDomain=network_engine_domain  SubClassName=ps_input  LeftPortType=input  RightPortType=output  PseudoPeriodic=off  Frequencies=[]  NoiseDistribution=none  NoiseParameters=[]  Unit=N*m  AffineConversion=off  FilteringAndDerivatives=zero  SimscapeFilterOrder=1  InputFilterTimeConstant=0.001  UdotUserProvided=1
  R : PMIOPort  Side=Right
  tag scope: trqDemand=global
  wires:
  Constant1/1 -> Simulink-PS Converter/1, [trqDemand]
  connections:
  Simulink-PS Converter/RConn1 -- R/RConn1

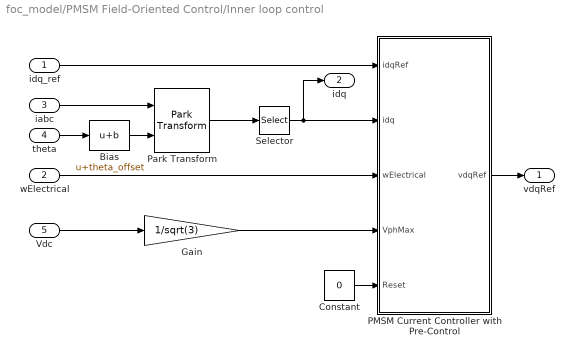
== system foc_model/PMSM Field-Oriented Control/Inner loop control ==
  idq_ref : Inport
  wElectrical : Inport  Port=2
  iabc : Inport  Port=3
  theta : Inport  Port=4
  Vdc : Inport  Port=5
  Bias : Bias  Bias=theta_offset
  Constant : Constant  Value=0  SampleTime=-1
  Gain : Gain  Gain=1/sqrt(3)
  PMSM Current Controller with Pre-Control : Subsystem  AncestorBlock=eePmsmCurrentController/PMSM Current Controller with Pre-Control  LoadFcn=ee_sli_rtmsupport( 'loadfcn', gcbh );  mask(PMSM Current Controller with Pre-Control){Kp_id=Kp_id, Ki_id=Ki_id, Kaw_id=Kaw_id, Kp_iq=Kp_iq, Ki_iq=Ki_iq, Kaw_iq=Kaw_iq, Ts=Tsc, Tsd=0.001, AxisPrio=Q-axis, ActZC=off, ActFF=on, idVect=idVect, iqVect=iqVect, LdMatrix=LdMatrix, LqMatrix=LqMatrix, psimMatrix=psimMatrix}
      mask prompts: Kp_id "physmod:ee:library:comments:control:eePmsmCurrentController:DaxisCurrentProportionalGain_MP"; Ki_id "physmod:ee:library:comments:control:eePmsmCurrentController:DaxisCurrentIntegralGain_MP"; Kaw_id "physmod:ee:library:comments:control:eePmsmCurrentController:DaxisCurrentAntiwindupGain_MP"; Kp_iq "physmod:ee:library:comments:control:eePmsmCurrentController:QaxisCurrentProportionalGain_MP"; Ki_iq "physmod:ee:library:comments:control:eePmsmCurrentController:QaxisCurrentIntegralGain_MP"; Kaw_iq "physmod:ee:library:comments:control:eePmsmCurrentController:QaxisCurrentAntiwindupGain_MP"; Ts "physmod:ee:library:comments:control:eePmsmCurrentController:SampleTime1ForInherited_MP"; Tsd "physmod:ee:library:comments:control:eePmsmCurrentController:DiscretizationSampleTime_MP"; AxisPrio "physmod:ee:library:comments:control:eePmsmCurrentController:AxisPrioritization_MP"; ActZC "physmod:ee:library:comments:control:eePmsmCurrentController:EnableZeroCancellation_MP"; ActFF "physmod:ee:library:comments:control:eePmsmCurrentController:EnablePrecontrolVoltage_MP"; idVect "physmod:ee:library:comments:control:eePmsmCurrentController:DaxisCurrentVectorIdA_MP"; iqVect "physmod:ee:library:comments:control:eePmsmCurrentController:QaxisCurrentVectorIqA_MP"; LdMatrix "physmod:ee:library:comments:control:eePmsmCurrentController:LdMatrixLdidiqH_MP"; LqMatrix "physmod:ee:library:comments:control:eePmsmCurrentController:LqMatrixLqidiqH_MP"; psimMatrix "physmod:ee:library:comments:control:eePmsmCurrentController:PermanentMagnetFluxLinkageMatrixPMidiqWb_MP"
      mask help: physmod:ee:library:comments:control:eePmsmCurrentController:PMSMCurrentControllerWithPreControl_MD
      mask init:
      | [Tsd, numZC_id, denZC_id, numZC_iq, denZC_iq] = ee.mask.initializePmsmCurrentController(ActZC,Ts,Tsd,Kp_id,Ki_id,Kp_iq,Ki_iq);
      | 
      | if length(idVect) < 2            
      | 	error(message('physmod:simscape:compiler:patterns:checks:LengthGreaterThanOrEqual',getString(message('physmod:ee:library:comments:control:eePmsmCurrentController:DaxisCurrentVectorIdA_MP')), '2'));            
      | end
      | if ~all(diff(idVect) > 0)            
      | 	error(message('physmod:simscape:compiler:patterns:checks:StrictlyAscendingVec',getString(message('physmod:ee:library:comments:control:eePmsmCurrentController:DaxisCurrentVectorIdA_MP'))));            
      | end
      | if length(iqVect) < 2            
      | 	error(message('physmod:simscape:compiler:patterns:checks:LengthGreaterThanOrEqual',getString(message('physmod:ee:library:comments:control:eePmsmCurrentController:QaxisCurrentVectorIqA_MP')), '2'));            
      | end
      | if ~all(diff(iqVect) > 0)            
      | 	error(message('physmod:simscape:compiler:patterns:checks:StrictlyAscendingVec',getString(message('physmod:ee:library:comments:control:eePmsmCurrentController:QaxisCurrentVectorIqA_MP'))));            
      | end
      | if ~all(size(LdMatrix) == [length(idVect), length(iqVect)])            
      | 	error(message('physmod:simscape:compiler:patterns:checks:Size2DEqual',getString(message('physmod:ee:library:comments:control:eePmsmCurrentController:LdMatrixLdidiqH_MP')), getString(message('physmod:ee:library:comments:control:eePmsmCurrentController:DaxisCurrentVectorIdA_MP')), getString(message('physmod:ee:library:comments:control:eePmsmCurrentController:QaxisCurrentVectorIqA_MP'))));            
      | end
      | if ~all(size(LqMatrix) == [length(idVect), length(iqVect)])            
      | 	error(message('physmod:simscape:compiler:patterns:checks:Size2DEqual',getString(message('physmod:ee:library:comments:control:eePmsmCurrentController:LqMatrixLqidiqH_MP')), getString(message('physmod:ee:library:comments:control:eePmsmCurrentController:DaxisCurrentVectorIdA_MP')), getString(message('physmod:ee:library:comments:control:eePmsmCurrentController:QaxisCurrentVectorIqA_MP'))));            
      | end
      | if ~all(size(psimMatrix) == [length(idVect), length(iqVect)])            
      | 	error(message('physmod:simscape:compiler:patterns:checks:Size2DEqual',getString(message('physmod:ee:library:comments:control:eePmsmCurrentController:PermanentMagnetFluxLinkageMatrixPMidiqWb_MP')), getString(message('physmod:ee:library:comments:control:eePmsmCurrentController:DaxisCurrentVectorIdA_MP')), getString(message('physmod:ee:library:comments:control:eePmsmCurrentController:QaxisCurrentVectorIqA_MP'))));            
      | end
      settings: CopyFcn=ee_sli_rtmsupport( 'copyfcn', gcbh );  DeleteFcn=ee_sli_rtmsupport( 'deletefcn', gcbh );  ModelCloseFcn=ee_sli_rtmsupport( 'modelclosefcn', gcbh );  PostSaveFcn=ee_sli_rtmsupport( 'postsavefcn', gcbh );  PreCopyFcn=ee_sli_rtmsupport( 'precopyfcn', gcbh );  OpenFcn=ee_sli_rtmsupport( 'openfcn', gcbh );  CloseFcn=ee_sli_rtmsupport( 'closefcn', gcbh );  PreDeleteFcn=ee_sli_rtmsupport( 'predeletefcn', gcbh );
      mask Help: web(nesl_help(gcbh))
      mask Callback Ts: ee.mask.callbackZeroCancellation(gcb);
      mask TypeOptions AxisPrio: d-q Voltage Limiter/AxisPrio
      mask Callback ActZC: ee.mask.callbackZeroCancellation(gcb);
      mask DialogControl Container3 Prompt: physmod:ee:library:comments:control:eePmsmCurrentController:tab_ControlParameters
      mask DialogControl Kp_id Prompt: D-axis current proportional gain
      mask DialogControl Ki_id Prompt: D-axis current integral gain
      mask DialogControl Kaw_id Prompt: D-axis current anti-windup gain
      mask DialogControl Kp_iq Prompt: Q-axis current proportional gain
      mask DialogControl Ki_iq Prompt: Q-axis current integral gain
      mask DialogControl Kaw_iq Prompt: Q-axis current anti-windup gain
      mask DialogControl Ts Prompt: Sample time (-1 for inherited)
      mask DialogControl Tsd Prompt: Discretization sample time
      mask DialogControl AxisPrio Prompt: Axis prioritization
      mask DialogControl ActZC Prompt: Enable zero cancellation
      mask DialogControl ActFF Prompt: Enable pre-control voltage
      mask DialogControl Container4 Prompt: physmod:ee:library:comments:control:eePmsmCurrentController:tab_PreControlParameters
      mask DialogControl idVect Prompt: D-axis current vector, id (A)
      mask DialogControl iqVect Prompt: Q-axis current vector, iq (A)
      mask DialogControl LdMatrix Prompt: Ld matrix, Ld(id,iq), (H)
      mask DialogControl LqMatrix Prompt: Lq matrix, Lq(id,iq), (H)
      mask DialogControl psimMatrix Prompt: Permanent magnet flux linkage matrix, PM(id,iq), (Wb)
  Park Transform : eeTransforms/Park Transform  AxisAlignment=Q-axis  PowerInvariant=off
  Selector : Selector  InputPortWidth=3  IndexOptions=Index vector (dialog)  Indices=[1 2]  OutputSizes=1
  vdqRef : Outport  VectorParamsAs1DForOutWhenUnconnected=off
  idq : Outport  Port=2  VectorParamsAs1DForOutWhenUnconnected=off
  wires:
  Bias/1 -> Park Transform/2
  PMSM Current Controller with Pre-Control/1(vdqRef) -> vdqRef/1
  Vdc/1 -> Gain/1
  wElectrical/1 -> PMSM Current Controller with Pre-Control/3(wElectrical)
  theta/1 -> Bias/1
  iabc/1 -> Park Transform/1
  idq_ref/1 -> PMSM Current Controller with Pre-Control/1(idqRef)
  Park Transform/1 -> Selector/1
  Gain/1 -> PMSM Current Controller with Pre-Control/4(VphMax)
  Selector/1 -> idq/1, PMSM Current Controller with Pre-Control/2(idq)
  Constant/1 -> PMSM Current Controller with Pre-Control/5(Reset)

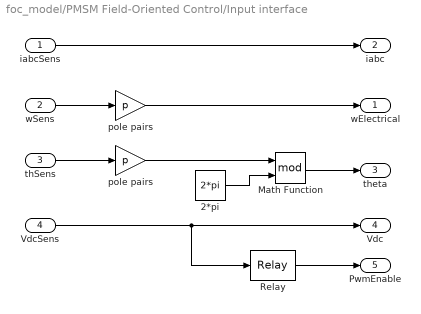
== system foc_model/PMSM Field-Oriented Control/Input interface ==
  iabcSens : Inport
  wSens : Inport  Port=2
  thSens : Inport  Port=3
  VdcSens : Inport  Port=4
  2*pi : Constant  Value=2*pi  SampleTime=Tsc
  Math Function : Math  Operator=mod  SignedPower=on  SaturateOnIntegerOverflow=on
  Relay : Relay  OnSwitchValue=Vdc_on  OffSwitchValue=0.5*Vdc_on
  pole pairs : Gain  Gain=p
  "pole pairs " : Gain  Gain=p
  wElectrical : Outport  VectorParamsAs1DForOutWhenUnconnected=off
  iabc : Outport  Port=2  VectorParamsAs1DForOutWhenUnconnected=off
  theta : Outport  Port=3  VectorParamsAs1DForOutWhenUnconnected=off
  Vdc : Outport  Port=4  VectorParamsAs1DForOutWhenUnconnected=off
  PwmEnable : Outport  Port=5  VectorParamsAs1DForOutWhenUnconnected=off
  wires:
  VdcSens/1 -> Vdc/1, Relay/1
  Relay/1 -> PwmEnable/1
  Math Function/1 -> theta/1
  2*pi/1 -> Math Function/2
  "pole pairs "/1 -> Math Function/1
  iabcSens/1 -> iabc/1
  wSens/1 -> pole pairs/1
  thSens/1 -> "pole pairs "/1
  pole pairs/1 -> wElectrical/1
